simulink model "model_one_upgrade1"  (R2025b)
settings: Solver=VariableStepAuto  StartTime=0.0  StopTime=600  RelTol=1e-3
undefined symbols (not defined in the file or in its folder): battery_builder_rtmsupport, gcbh
libraries: nesl_utility x9, fl_lib x8, Batteries_Pack_lib x2, autolibshared x1, mqttlib x1, batt_lib x1, BatteryBalancing x1
(part 1 of 2)
settings Model: PacingRate=11  Creator=DELL  LastModifiedBy=my802
settings DebuggingCC: AlgebraicLoopMsg=none

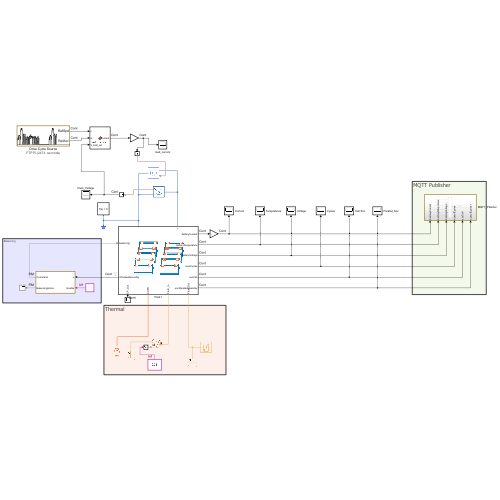
[thumbnail: Simulink's stored preview of the top-level diagram]
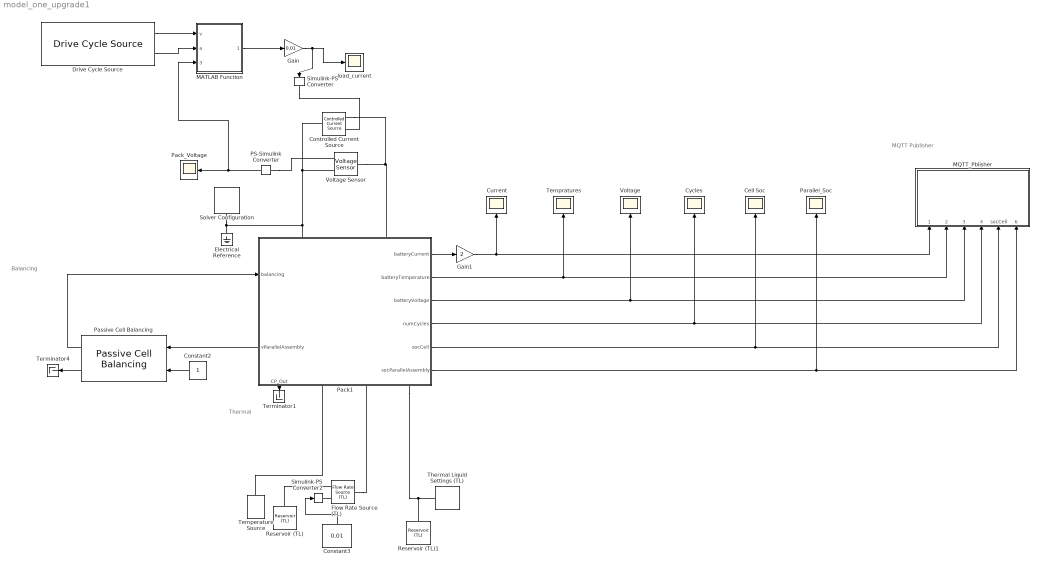
== system model_one_upgrade1 ==
  note: MQTT Publisher
  note: Balancing
  note: Thermal
  Cell Soc : Scope
      settings: ActiveDisplayYMinimum=0.546688606760402  ActiveDisplayYMaximum=0.829439556546784  DataLoggingVariableName=ScopeData6
  Constant2 : Constant
  Constant3 : Constant  Value=0.01
  Controlled Current Source : fl_lib/Electrical/Electrical Sources/Controlled Current Source
  Current : Scope
      settings: ActiveDisplayYMinimum=-32.846312604360023  ActiveDisplayYMaximum=11.836410191491415
  Cycles : Scope
      settings: ActiveDisplayYMinimum=-0.0029468529954673551  ActiveDisplayYMaximum=0.02652167582790381  DataLoggingVariableName=ScopeData9
  Drive Cycle Source : autolibshared/Drive Cycle Source  cycleVar=FTP75  fileVar=cycleFTP75.mat  tfinal="2474  seconds"  cycleRepeat=off  outAccPort=on  outGearPort=off  gearList=No gear data  t_wot1=5  xdot_woto=0  xdot_wot1=30  t_wot2=20  xdot_wot2=0  t_wotend=30  srcUnit=m/s  outUnit=m/s  srcAccUnit=m/s/s  outAccUnit=m/s^2  dt=0  aMode=1  faultOption=off  velBnd=2  velBndUnit=mph  inUnit=m/s  timeBnd=1  failOption=off  stopSim=off  maxFaultCnt=10  maxFaultTime=2  maxTotFaultTime=15  traceOption=off  dtTrace=1  traceWindow=10  lastDCname=FTP75  lastOutUnit=mph  lastDT=0  lastTB=1  lastSB=2  forceCalcBound=off
  Electrical Reference : fl_lib/Electrical/Electrical Elements/Electrical Reference
  Flow Rate Source (TL) : fl_lib/Thermal Liquid/Sources/Flow Rate Source (TL)  source_type=foundation.enum.constant_controlled.controlled  flow_type=foundation.enum.mass_volumetric_flow.mass  mass_flow=0 kg/s  volumetric_flow=0 m^3/s  power_spec=foundation.enum.power_spec.isentropic  area=0.01 m^2
  Gain : Gain  Gain=0.01
  Gain1 : Gain  Gain=2
  MATLAB Function : MATLAB Function  TreatAsAtomicUnit=on
  MQTT_Pblisher : Subsystem
  PS-Simulink Converter : nesl_utility/PS-Simulink Converter  PhysicalDomain=network_engine_domain  SubClassName=ps_output  LeftPortType=input  RightPortType=output  PseudoPeriodic=off  Frequencies=[]  VectorFormat=inherit  Unit=inherit  AffineConversion=off
  Pack1 : Subsystem  LoadFcn=battery_builder_rtmsupport('loadfcn',gcbh);
      settings: CopyFcn=battery_builder_rtmsupport('copyfcn',gcbh);  PreCopyFcn=battery_builder_rtmsupport('precopyfcn',gcbh);  PreDeleteFcn=battery_builder_rtmsupport('predeletefcn',gcbh);  PortSchema="{\"entries\":[{\"content\":{\"sides\":[{\"content\":{\"connectorIds\":[\"LConn1\",\"LConn2\"]},\"type\":\"ConnectorPlacement.EquallySpacedRectSide\",\"uuid\":\"55a5794a-5ecf-4a83-8d77-34dfd6810a2f\"},{\"content\":{\"connectorIds\":[\"Out1\",\"RConn1\",\"RConn2\",\"RConn3\"],\"side\":\"RIGHT\"},\"type\":\"ConnectorPlacement.EquallySpacedRectSide\",\"uuid\":\"d8a6a3e5-5c93-4739-9223-e5221a5356c5\"},{\"content\":{\"connectorIds\":[\"In1\",\"Out8\"],\"side\":\"TOP\"},\"type\":\"ConnectorPlacement.EquallySpacedRectSide\",\"uuid\":\"e9ee7270-cbe6-4e4f-8234-b65e137cf24d\"},{\"content\":{\"connectorIds\":[\"Out2\",\"Out3\",\"Out4\",\"Out5\",\"Out6\",\"Out7\"],\"side\":\"BOTTOM\"},\"type\":\"ConnectorPlacement.EquallySpacedRectSide\",\"uuid\":\"56854e54-bf02-4170-8eb1-11b06e8960f7\"}]},\"type\":\"ConnectorPlacement.EquallySpacedConnector\",\"uuid\":\"e45f6c19-a0f4-4da6-938a-e1e4a4f7821b\"}],\"packageUris\":[\"http://schema.mathworks.com/mf0/Connector/R2020b\"],\"version\":\"1.0\"}"
      mask Display: image('$imagefile')
  Pack_Voltage : Scope
      settings: ActiveDisplayYMinimum=11.015291198745329  ActiveDisplayYMaximum=17.499738477567043
  Parallel_Soc : Scope
      settings: ActiveDisplayYMinimum=0.548996443495374  ActiveDisplayYMaximum=0.8458849402649733  DataLoggingVariableName=ScopeData8
  Passive Cell Balancing : BatteryBalancing/Passive Cell Balancing  Threshold=0.2  HysteresisBand=0  Td_on=1  Td_off=1  Ts=-1  dataType=double
      settings: LibrarySourceBlock=batt_sl_lib/Cell Balancing/Passive Cell Balancing
  Reservoir (TL) : fl_lib/Thermal Liquid/Elements/Reservoir (TL)  pressure_spec=foundation.enum.pressure_spec.atmospheric  reservoir_pressure=0.101325 MPa  reservoir_temperature=293.15 K  area=0.01 m^2
  Reservoir (TL)1 : fl_lib/Thermal Liquid/Elements/Reservoir (TL)  pressure_spec=foundation.enum.pressure_spec.atmospheric  reservoir_pressure=0.101325 MPa  reservoir_temperature=293.15 K  area=0.01 m^2
  Simulink-PS Converter : nesl_utility/Simulink-PS Converter  PhysicalDomain=network_engine_domain  SubClassName=ps_input  LeftPortType=input  RightPortType=output  PseudoPeriodic=off  Frequencies=[]  NoiseDistribution=none  NoiseParameters=[]  Unit=1  AffineConversion=off  FilteringAndDerivatives=provide  SimscapeFilterOrder=1  InputFilterTimeConstant=0.001  UdotUserProvided=0
  Simulink-PS Converter2 : nesl_utility/Simulink-PS Converter  PhysicalDomain=network_engine_domain  SubClassName=ps_input  LeftPortType=input  RightPortType=output  PseudoPeriodic=off  Frequencies=[]  NoiseDistribution=none  NoiseParameters=[]  Unit=1  AffineConversion=off  FilteringAndDerivatives=provide  SimscapeFilterOrder=1  InputFilterTimeConstant=0.001  UdotUserProvided=0
  Solver Configuration : nesl_utility/Solver Configuration  PhysicalDomain=network_engine_domain  SubClassName=solver  LeftPortType=input  RightPortType=generic  Tones=[]  Harmonics=[]  SimulateNoise=off  Profile=off  UseLocalSampling=off  EnableSwitchedLinearOptims=on  FrequencyDomain=off  UseCCode=off  RelTol=0.001  AbsTol=0.001  MinStep=1e-09  ToWorkspace=off  RevertToSquareIcSolve=off  NumHomotopyIterations=100  PhasorMode=off  PhasorModeNumHarmonics=1  ConsistencySolver=NEWTON_XTOL_AFTER_FTOL  IndexReductionMethod=DerivativeReplacement  DoDC=off  ResidualTolerance=1e-09  ConsistencyTolSource=GLOBAL  ConsistencyAbsTol=0.001  ConsistencyRelTol=0.001  ConsistencyTolFactor=0.001  UseLocalSolver=off  LocalSolverChoice=NE_BACKWARD_EULER_ADVANCER  ResolveIndetEquations=on  FunctionEvalNumThread=1  LocalSolverSampleTime=0.001  DoFixedCost=off  MaxNonlinIter=3  MaxModeIter=2  ComputeImpulses=off  ImpulseIterations=2  LinearAlgebra=auto  LinearAlgebraNumThread=0  EquationFormulation=NE_TIME_EF  DelaysMemoryBudget=1024  AutomaticFiltering=on  FilteringTimeConstant=0.001  PartitionStorageMethod=AS_NEEDED  PartitionMemoryBudget=1024  PartitionMethod=ROBUST  MultibodyUseLocalSolver=off  MultibodyLocalSolverChoice=ODE1  MultibodyLocalSolverSampleTime=0.001
  Temperature Source : fl_lib/Thermal/Thermal Sources/Temperature Source  temperature=298.15 K
  Tempratures : Scope
      settings: ActiveDisplayYMinimum=297.03118131262454  ActiveDisplayYMaximum=305.45250178286375  DataLoggingVariableName=ScopeData4
  Terminator1 : Terminator
  Terminator4 : Terminator
  Thermal Liquid Settings (TL) : fl_lib/Thermal Liquid/Utilities/Thermal Liquid Settings (TL)  table_dimensions=foundation.enum.table_dimensions_TL.two_dimensional  T_TLU=[273.1600 : 10 : 373.16]' K  p_TLU=[0.01, 0.1, 5 : 5 : 50] MPa  p_atm=0.101325 MPa  pT_region_flag=foundation.enum.pT_region_TL.min_max  T_min=273.16 K  T_max=373.16 K  p_min=0.01 MPa  p_max=50 MPa  T_min_1D=273.16 K  T_max_1D=373.16 K  p_min_1D=0.01 MPa  p_max_1D=50 MPa  pT_validity_TLU=[1, 1, 1, 1, 1, 1, 1, 1, 1, 1, 1, 1; 1, 1, 1, 1, 1, 1, 1, 1, 1, 1, 1, 1; 1, 1, 1, 1, 1, 1, 1, 1, 1, 1, 1, 1; 1, 1, 1, 1, 1, 1, 1, 1, 1, 1, 1, 1; 1, 1, 1, 1, 1, 1, 1, 1, 1, 1, 1, 1; 0, 1, 1, 1, 1, 1, 1, 1, 1, 1, 1, 1; 0, 1, 1, 1, 1, 1, 1, 1, 1, 1, 1, 1; 0, 1, 1, 1, 1, 1, 1, 1, 1, 1, 1, 1; 0, 1, 1, 1, 1, 1, 1, 1, 1, 1, 1, 1; 0, 1, 1, 1, 1, 1, 1, 1, 1, 1, 1, 1; 0, 0, 1, 1, 1, 1, 1, 1, 1, 1, 1, 1]  properties_range_check=simscape.enum.assert.action.error  rho_parameterization_2D=foundation.enum.rho_parameterization_2D.rho_beta_alpha  rho_parameterization_1D=foundation.enum.rho_parameterization_1D.rho_vector  rho_TLU=[999.7973, 999.8431, 1002.3216, 1004.8218, 1007.293, 1009.7358, 1012.1506, 1014.5379, 1016.8979, 1019.2311, 1021.538, 1023.8188; 999.6579, 999.7009, 1002.0303, 1004.382, 1006.7084, 1009.0101, 1011.2874, 1013.5407, 1015.7703, 1017.9766, 1020.1599, 1022.3206; 998.1632, 998.2045, 1000.4375, 1002.6924, 1004.9239, 1007.1324, 1009.3183, 1011.4819, 1013.6236, 1015.7438, 1017.8428, 1019.921; 995.6057, 995.6458, 997.8186, 1000.0128, 1002.1841, 1004.3332, 1006.4603, 1008.566, 1010.6505, 1012.7144, 1014.758, 1016.7815; 992.1724, 992.2119, 994.3513, 996.5113, 998.6484, 1000.7633, 1002.8563, 1004.928, 1006.9788, 1009.009, 1011.0192, 1013.0097; 988.02, 988.0299, 990.1568, 992.3035, 994.4268, 996.5273, 998.6056, 1000.6622, 1002.6976, 1004.7123, 1006.7067, 1008.6813; 983.18, 983.1901, 985.3217, 987.4721, 989.5983, 991.7008, 993.7803, 995.8374, 997.8726, 999.8864, 1001.8795, 1003.8522; 977.75, 977.7583, 979.9094, 982.0783, 984.2216, 986.34, 988.4343, 990.505, 992.5529, 994.5786, 996.5825, 998.5654; 971.77, 971.7836, 973.9673, 976.1678, 978.3409, 980.4876, 982.6087, 984.7049, 986.7768, 988.8254, 990.8511, 992.8545; 965.26, 965.3023, 967.5311, 969.7753, 971.9901, 974.1764, 976.3354, 978.4676, 980.5741, 982.6556, 984.7129, 986.7465; 958.62, 958.6315, 960.627, 962.9267, 965.1944, 967.4314, 969.6387, 971.8173, 973.9681, 976.0921, 978.19, 980.2628] kg/m^3  beta_TLU=[1.9649, 1.9654, 1.9929, 2.0213, 2.0499, 2.0787, 2.1078, 2.1372, 2.1668, 2.1966, 2.2268, 2.2572; 2.0913, 2.0918, 2.1191, 2.1471, 2.1752, 2.2036, 2.2322, 2.261, 2.2899, 2.3191, 2.3485, 2.3781; 2.1786, 2.1791, 2.2067, 2.235, 2.2634, 2.2919, 2.3206, 2.3494, 2.3784, 2.4075, 2.4367, 2.4661; 2.2332, 2.2337, 2.2619, 2.2908, 2.3197, 2.3487, 2.3778, 2.407, 2.4363, 2.4657, 2.4951, 2.5246; 2.26, 2.2605, 2.2895, 2.3191, 2.3487, 2.3784, 2.4081, 2.4378, 2.4675, 2.4973, 2.5272, 2.5571; 2.2638, 2.2638, 2.2936, 2.324, 2.3544, 2.3848, 2.4151, 2.4455, 2.4758, 2.5062, 2.5365, 2.5669; 2.2472, 2.2472, 2.2779, 2.3092, 2.3403, 2.3715, 2.4025, 2.4336, 2.4646, 2.4955, 2.5264, 2.5573; 2.214, 2.214, 2.2455, 2.2776, 2.3096, 2.3415, 2.3733, 2.405, 2.4367, 2.4683, 2.4998, 2.5313; 2.1668, 2.1668, 2.1992, 2.2321, 2.2649, 2.2976, 2.3301, 2.3626, 2.3949, 2.4272, 2.4593, 2.4914; 2.1081, 2.1081, 2.1413, 2.175, 2.2086, 2.2421, 2.2754, 2.3085, 2.3415, 2.3744, 2.4072, 2.4399; 2.0494, 2.0494, 2.0739, 2.1084, 2.1428, 2.177, 2.211, 2.2449, 2.2786, 2.3121, 2.3455, 2.3788] GPa  alpha_TLU=1e-4 * [-.679, -.676, -.49, -.307, -.13, .041, .206, .365, .519, .668, .811, .949; .878, .881, .998, 1.114, 1.227, 1.337, 1.445, 1.549, 1.651, 1.75, 1.846, 1.939; 2.068, 2.069, 2.141, 2.213, 2.283, 2.352, 2.42, 2.486, 2.551, 2.614, 2.676, 2.736; 3.034, 3.035, 3.074, 3.113, 3.152, 3.191, 3.229, 3.267, 3.305, 3.341, 3.377, 3.413; 3.855, 3.856, 3.87, 3.884, 3.899, 3.914, 3.93, 3.946, 3.961, 3.977, 3.993, 4.009; 4.578, 4.578, 4.572, 4.566, 4.562, 4.558, 4.555, 4.552, 4.55, 4.549, 4.548, 4.547; 5.233, 5.233, 5.209, 5.186, 5.165, 5.144, 5.125, 5.107, 5.09, 5.074, 5.059, 5.045; 5.84, 5.84, 5.801, 5.762, 5.725, 5.691, 5.657, 5.625, 5.595, 5.566, 5.538, 5.512; 6.414, 6.414, 6.36, 6.307, 6.256, 6.208, 6.161, 6.117, 6.074, 6.033, 5.994, 5.956; 6.967, 6.967, 6.898, 6.831, 6.766, 6.705, 6.646, 6.589, 6.535, 6.482, 6.432, 6.384; 7.519, 7.519, 7.423, 7.342, 7.264, 7.189, 7.118, 7.049, 6.983, 6.92, 6.859, 6.8] 1/K  rho_TLU_2=[999.7973, 999.8431, 1002.3216, 1004.8218, 1007.293, 1009.7358, 1012.1506, 1014.5379, 1016.8979, 1019.2311, 1021.538, 1023.8188; 999.6579, 999.7009, 1002.0303, 1004.382, 1006.7084, 1009.0101, 1011.2874, 1013.5407, 1015.7703, 1017.9766, 1020.1599, 1022.3206; 998.1632, 998.2045, 1000.4375, 1002.6924, 1004.9239, 1007.1324, 1009.3183, 1011.4819, 1013.6236, 1015.7438, 1017.8428, 1019.921; 995.6057, 995.6458, 997.81864, 1000.0128, 1002.1841, 1004.3332, 1006.4603, 1008.566, 1010.6505, 1012.7144, 1014.758, 1016.7815; 992.1724, 992.2119, 994.3513, 996.5113, 998.6484, 1000.7633, 1002.8563, 1004.928, 1006.9788, 1009.009, 1011.0192, 1013.0097; 988.02, 988.0299, 990.1568, 992.3035, 994.4268, 996.5273, 998.6056, 1000.6622, 1002.6976, 1004.7123, 1006.7067, 1008.6813; 983.18, 983.1901, 985.3217, 987.4721, 989.5983, 991.7008, 993.7803, 995.8374, 997.8726, 999.8864, 1001.8795, 1003.8522; 977.75, 977.7583, 979.9094, 982.0783, 984.2216, 986.34, 988.4343, 990.505, 992.5529, 994.5786, 996.5825, 998.5654; 971.77, 971.7836, 973.9673, 976.1678, 978.3409, 980.4876, 982.6087, 984.7049, 986.7768, 988.8254, 990.8511, 992.8545; 965.26, 965.3023, 967.5311, 969.7753, 971.9901, 974.1764, 976.3354, 978.4676, 980.5741, 982.6556, 984.7129, 986.7465; 958.62, 958.6315, 960.627, 962.9267, 965.1944, 967.4314, 969.6387, 971.8173, 973.9681, 976.0921, 978.19, 980.2628] kg/m^3  rho_ref_3=998.21 kg/m^3  T_ref_3=293.16 K  p_ref_3=0.101325 MPa  beta_const_3=2.1791 GPa  alpha_const_3=2.0691e-4 1/K  rho_TLU_4=[999.84; 999.7; 998.2; 995.65; 992.21; 988.03; 983.19; 977.76; 971.78; 965.3; 958.8] kg/m^3  beta_const_4=2.1791 GPa  p_ref_4=0.101325 MPa  rho_ref_5=998.21 kg/m^3  T_ref_5=293.16 K  p_ref_5=0.101325 MPa  beta_const_5=2.1791 GPa  alpha_const_5=2.0691e-4 1/K  u_parameterization_2D=foundation.enum.u_parameterization_2D.u_cp  u_parameterization_1D=foundation.enum.u_parameterization_1D.u  u_TLU=[.0002, .0018, .086, .1588, .219, .267, .3034, .3288, .3436, .3483, .3435, .3294; 42.062, 42.06, 41.935, 41.804, 41.668, 41.527, 41.382, 41.233, 41.081, 40.924, 40.763, 40.599; 83.953, 83.948, 83.651, 83.349, 83.049, 82.749, 82.451, 82.153, 81.856, 81.56, 81.265, 80.971; 125.77, 125.76, 125.31, 124.86, 124.41, 123.97, 123.53, 123.1, 122.68, 122.25, 121.84, 121.42; 167.57, 167.56, 166.96, 166.37, 165.79, 165.21, 164.65, 164.09, 163.54, 163, 162.46, 161.94; 209.36, 209.36, 208.63, 207.9, 207.19, 206.48, 205.79, 205.11, 204.45, 203.79, 203.14, 202.5; 251.19, 251.19, 250.33, 249.47, 248.62, 247.79, 246.98, 246.18, 245.39, 244.62, 243.86, 243.12; 293.06, 293.06, 292.07, 291.07, 290.1, 289.14, 288.2, 287.28, 286.38, 285.49, 284.62, 283.77; 334.99, 334.99, 333.86, 332.73, 331.63, 330.54, 329.48, 328.44, 327.41, 326.41, 325.43, 324.46; 377, 377, 375.73, 374.46, 373.22, 372, 370.81, 369.64, 368.5, 367.38, 366.27, 365.19; 419.01, 419.01, 417.69, 416.27, 414.89, 413.54, 412.21, 410.91, 409.64, 408.4, 407.17, 405.98] kJ/kg  cp_TLU=[4.2199, 4.2194, 4.1957, 4.1726, 4.1508, 4.13, 4.1103, 4.0916, 4.0738, 4.0569, 4.0408, 4.0254; 4.1955, 4.1951, 4.1769, 4.1592, 4.1422, 4.1259, 4.1103, 4.0954, 4.0812, 4.0676, 4.0545, 4.0421; 4.1843, 4.184, 4.169, 4.1543, 4.1401, 4.1264, 4.1133, 4.1007, 4.0885, 4.0768, 4.0656, 4.0548; 4.1801, 4.1798, 4.1667, 4.1538, 4.1413, 4.1293, 4.1177, 4.1064, 4.0956, 4.0851, 4.075, 4.0653; 4.1796, 4.1794, 4.1675, 4.1558, 4.1444, 4.1334, 4.1227, 4.1123, 4.1023, 4.0926, 4.0832, 4.0741; 4.1813, 4.1813, 4.1702, 4.1592, 4.1484, 4.138, 4.1279, 4.1181, 4.1086, 4.0993, 4.0903, 4.0816; 4.185, 4.185, 4.1742, 4.1636, 4.1532, 4.1432, 4.1334, 4.1239, 4.1146, 4.1056, 4.0969, 4.0884; 4.1901, 4.1901, 4.1795, 4.169, 4.1588, 4.1489, 4.1393, 4.1299, 4.1207, 4.1118, 4.1032, 4.0947; 4.1968, 4.1968, 4.1862, 4.1757, 4.1655, 4.1555, 4.1458, 4.1364, 4.1273, 4.1183, 4.1096, 4.1012; 4.2052, 4.2052, 4.1944, 4.1837, 4.1733, 4.1632, 4.1534, 4.1438, 4.1345, 4.1255, 4.1166, 4.108; 4.2136, 4.2136, 4.2045, 4.1935, 4.1828, 4.1724, 4.1623, 4.1524, 4.1429, 4.1335, 4.1245, 4.1157] kJ/(K*kg)  u_TLU_2=[.0002, .0018, .086, .1588, .219, .267, .3034, .3288, .3436, .3483, .3435, .3294; 42.062, 42.06, 41.935, 41.804, 41.668, 41.527, 41.382, 41.233, 41.081, 40.924, 40.763, 40.599; 83.953, 83.948, 83.651, 83.349, 83.049, 82.749, 82.451, 82.153, 81.856, 81.56, 81.265, 80.971; 125.77, 125.76, 125.31, 124.86, 124.41, 123.97, 123.53, 123.1, 122.68, 122.25, 121.84, 121.42; 167.57, 167.56, 166.96, 166.37, 165.79, 165.21, 164.65, 164.09, 163.54, 163, 162.46, 161.94; 209.36, 209.36, 208.63, 207.9, 207.19, 206.48, 205.79, 205.11, 204.45, 203.79, 203.14, 202.5; 251.19, 251.19, 250.33, 249.47, 248.62, 247.79, 246.98, 246.18, 245.39, 244.62, 243.86, 243.12; 293.06, 293.06, 292.07, 291.07, 290.1, 289.14, 288.2, 287.28, 286.38, 285.49, 284.62, 283.77; 334.99, 334.99, 333.86, 332.73, 331.63, 330.54, 329.48, 328.44, 327.41, 326.41, 325.43, 324.46; 377, 377, 375.73, 374.46, 373.22, 372, 370.81, 369.64, 368.5, 367.38, 366.27, 365.19; 419.01, 419.01, 417.69, 416.27, 414.89, 413.54, 412.21, 410.91, 409.64, 408.4, 407.17, 405.98] kJ/kg  cp_TLU_3=[4.2199, 4.2194, 4.1957, 4.1726, 4.1508, 4.13, 4.1103, 4.0916, 4.0738, 4.0569, 4.0408, 4.0254; 4.1955, 4.1951, 4.1769, 4.1592, 4.1422, 4.1259, 4.1103, 4.0954, 4.0812, 4.0676, 4.0545, 4.0421; 4.1843, 4.184, 4.169, 4.1543, 4.1401, 4.1264, 4.1133, 4.1007, 4.0885, 4.0768, 4.0656, 4.0548; 4.1801, 4.1798, 4.1667, 4.1538, 4.1413, 4.1293, 4.1177, 4.1064, 4.0956, 4.0851, 4.075, 4.0653; 4.1796, 4.1794, 4.1675, 4.1558, 4.1444, 4.1334, 4.1227, 4.1123, 4.1023, 4.0926, 4.0832, 4.0741; 4.1813, 4.1813, 4.1702, 4.1592, 4.1484, 4.138, 4.1279, 4.1181, 4.1086, 4.0993, 4.0903, 4.0816; 4.185, 4.185, 4.1742, 4.1636, 4.1532, 4.1432, 4.1334, 4.1239, 4.1146, 4.1056, 4.0969, 4.0884; 4.1901, 4.1901, 4.1795, 4.169, 4.1588, 4.1489, 4.1393, 4.1299, 4.1207, 4.1118, 4.1032, 4.0947; 4.1968, 4.1968, 4.1862, 4.1757, 4.1655, 4.1555, 4.1458, 4.1364, 4.1273, 4.1183, 4.1096, 4.1012; 4.2052, 4.2052, 4.1944, 4.1837, 4.1733, 4.1632, 4.1534, 4.1438, 4.1345, 4.1255, 4.1166, 4.108; 4.2136, 4.2136, 4.2045, 4.1935, 4.1828, 4.1724, 4.1623, 4.1524, 4.1429, 4.1335, 4.1245, 4.1157] kJ/(K*kg)  u_TLU_4=[.0018; 42.06; 83.948; 125.76; 167.56; 209.36; 251.19; 293.06; 334.99; 377; 418.01] kJ/kg  cp_TLU_5=[4.2199; 4.1955; 4.1843; 4.1801; 4.1796; 4.1813; 4.185; 4.1901; 4.1968; 4.2052; 4.2136] kJ/(K*kg)  nu_TLU=[1.7917, 1.7914, 1.7763, 1.7615, 1.7473, 1.7338, 1.7208, 1.7085, 1.6967, 1.6854, 1.6747, 1.6645; 1.3061, 1.3059, 1.2986, 1.2914, 1.2845, 1.2779, 1.2716, 1.2656, 1.2598, 1.2543, 1.2491, 1.2441; 1.0032, 1.0032, .9995, .9959, .9924, .9891, .9859, .9829, .9801, .9774, .9748, .9724; .8006, .8005, .7987, .797, .7953, .7937, .7922, .7908, .7894, .7881, .787, .7859; .6577, .6577, .657, .6562, .6555, .6548, .6543, .6537, .6532, .6528, .6523, .652; .553, .553, .5529, .5527, .5526, .5525, .5524, .5524, .5524, .5524, .5524, .5525; .4739, .4739, .4741, .4743, .4745, .4747, .475, .4753, .4755, .4758, .4762, .4765; .4127, .4127, .4131, .4135, .4139, .4143, .4148, .4152, .4157, .4162, .4167, .4172; .3643, .3643, .3648, .3654, .3659, .3665, .367, .3676, .3682, .3688, .3694, .37; .3254, .3254, .3261, .3267, .3273, .328, .3286, .3293, .3299, .3306, .3312, .3319; .2866, .2866, .2945, .2952, .2959, .2965, .2972, .2979, .2986, .2993, .3, .3007] mm^2/s  nu_TLU_2=[1.7917; 1.3061; 1.0032; .8006; .6577; .553; .4739; .4127; .3643; .3254; .2866] mm^2/s  k_TLU=[561.04, 561.09, 563.8, 566.56, 569.32, 572.08, 574.82, 577.54, 580.24, 582.92, 585.57, 588.18; 580.02, 580.07, 582.45, 584.88, 587.32, 589.75, 592.18, 594.61, 597.02, 599.42, 601.8, 604.16; 598.44, 598.48, 600.73, 603.03, 605.33, 607.64, 609.94, 612.24, 614.54, 616.82, 619.1, 621.36; 615.48, 615.52, 617.73, 620, 622.26, 624.54, 626.81, 629.07, 631.34, 633.6, 635.85, 638.09; 630.6, 630.64, 632.87, 635.15, 637.44, 639.72, 642.01, 644.29, 646.57, 648.84, 651.11, 653.36; 643.61, 643.61, 645.88, 648.21, 650.53, 652.86, 655.18, 657.51, 659.82, 662.14, 664.44, 666.74; 654.39, 654.39, 656.73, 659.12, 661.5, 663.89, 666.27, 668.65, 671.02, 673.38, 675.74, 678.09; 663.13, 663.13, 665.54, 668, 670.46, 672.91, 675.36, 677.8, 680.24, 682.67, 685.09, 687.5; 670.02, 670.02, 672.51, 675.05, 677.59, 680.12, 682.64, 685.16, 687.67, 690.17, 692.66, 695.14; 675.27, 675.27, 677.85, 680.48, 683.11, 685.73, 688.34, 690.94, 693.53, 696.11, 698.68, 701.24; 680.52, 680.52, 681.77, 684.5, 687.22, 689.94, 692.64, 695.34, 698.02, 700.69, 703.35, 706] mW/(K*m)  k_TLU_2=[561.04; 580.02; 598.44; 615.48; 630.6; 643.61; 654.39; 663.13; 670.02; 675.27; 680.52] mW/(K*m)
  Voltage : Scope
      settings: ActiveDisplayYMinimum=3.7175558325329772  ActiveDisplayYMaximum=4.5563975278034681  DataLoggingVariableName=ScopeData5
  Voltage Sensor : fl_lib/Electrical/Electrical Sensors/Voltage Sensor
  load_current : Scope
      settings: ActiveDisplayYMinimum=-11.836404348489875  ActiveDisplayYMaximum=32.8462600292936  DataLoggingVariableName=ScopeData2
  wires:
  Constant2/1 -> Passive Cell Balancing/2
  Pack1/8(vParallelAssembly) -> Passive Cell Balancing/1
  Pack1/1(CP_Out) -> Terminator1/1
  Pack1/7(socParallelAssembly) -> Parallel_Soc/1, MQTT_Pblisher/6(numofCycles1)
  Pack1/5(numCycles) -> Cycles/1, MQTT_Pblisher/4(numofCycles)
  Pack1/4(batteryVoltage) -> Voltage/1, MQTT_Pblisher/3(batteryVoltage)
  Pack1/3(batteryTemperature) -> Tempratures/1, MQTT_Pblisher/2(batteryTemprature)
  Passive Cell Balancing/2 -> Terminator4/1
  Constant3/1 -> Simulink-PS Converter2/1
  Passive Cell Balancing/1 -> Pack1/1(balancing)
  Pack1/6(socCell) -> Cell Soc/1, MQTT_Pblisher/5(socCell)
  Drive Cycle Source/1 -> MATLAB Function/1(v)
  Drive Cycle Source/2 -> MATLAB Function/2(a)
  PS-Simulink Converter/1 -> Pack_Voltage/1, MATLAB Function/3(V_batt_act)
  MATLAB Function/1(Current) -> Gain/1
  Gain/1 -> Simulink-PS Converter/1, load_current/1
  Pack1/2(batteryCurrent) -> Gain1/1
  Gain1/1 -> MQTT_Pblisher/1(batteryCurrent), Current/1
  connections:
  Solver Configuration/RConn1 -- Voltage Sensor/RConn2 -- Controlled Current Source/LConn1 -- Pack1/LConn1 -- Electrical Reference/LConn1
  Reservoir (TL)/LConn1 -- Flow Rate Source (TL)/LConn1
  Flow Rate Source (TL)/RConn1 -- Pack1/RConn2
  Pack1/RConn3 -- Thermal Liquid Settings (TL)/RConn1 -- Reservoir (TL)1/LConn1
  Temperature Source/LConn1 -- Pack1/RConn1
  Simulink-PS Converter2/RConn1 -- Flow Rate Source (TL)/LConn2
  Voltage Sensor/LConn1 -- Controlled Current Source/RConn2 -- Pack1/LConn2
  PS-Simulink Converter/LConn1 -- Voltage Sensor/RConn1
  Simulink-PS Converter/RConn1 -- Controlled Current Source/RConn1

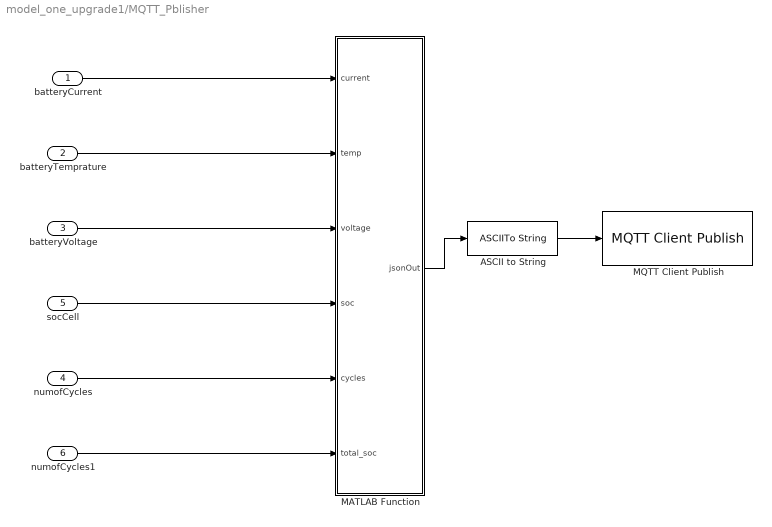
== system model_one_upgrade1/MQTT_Pblisher ==
  batteryCurrent : Inport
  batteryTemprature : Inport  Port=2
  batteryVoltage : Inport  Port=3
  numofCycles : Inport  Port=4
  socCell : Inport  Port=5
  numofCycles1 : Inport  Port=6
  ASCII to String : ASCIIToString
  MATLAB Function : MATLAB Function  TreatAsAtomicUnit=on
  MQTT Client Publish : mqttlib/MQTT Client Publish  RetainClient=MQTT_BROKER  ClientList=MQTT_BROKER  TopicsTable={ '1', 'Pack', '0', 'on' }  PublishOnDataChange=on  SampleTime=-1  TopicNames=Pack  NumTopics=1  IsLib=0  BlkName=MQTT Client Publish
  wires:
  batteryCurrent/1 -> MATLAB Function/1(current)
  batteryTemprature/1 -> MATLAB Function/2(temp)
  batteryVoltage/1 -> MATLAB Function/3(voltage)
  numofCycles/1 -> MATLAB Function/5(cycles)
  socCell/1 -> MATLAB Function/4(soc)
  MATLAB Function/1(jsonOut) -> ASCII to String/1
  ASCII to String/1 -> MQTT Client Publish/1
  numofCycles1/1 -> MATLAB Function/6(total_soc)

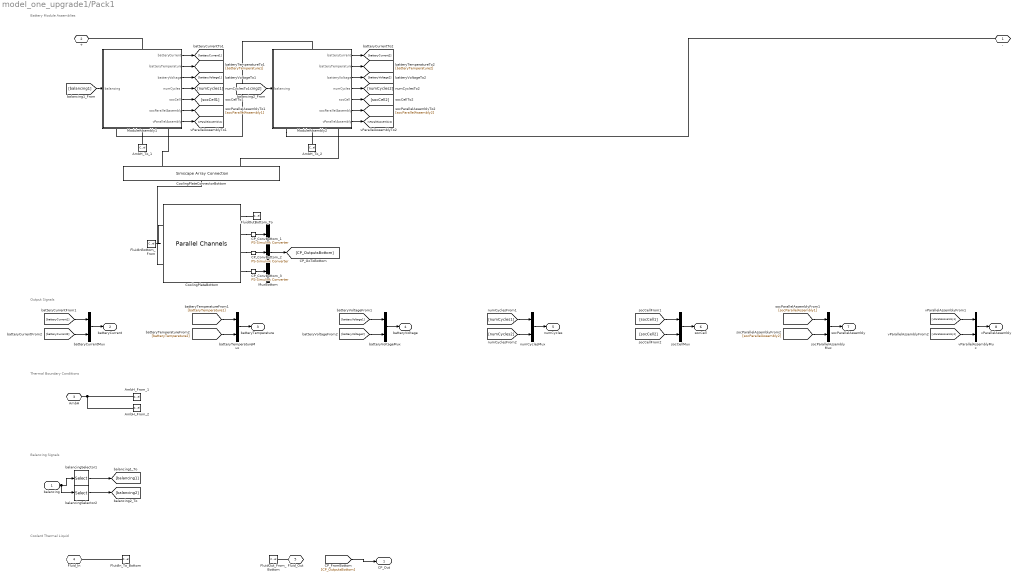
== system model_one_upgrade1/Pack1 ==
  note: Coolant Thermal Liquid
  note: Balancing Signals
  note: Thermal Boundary Conditions
  note: Output Signals
  note: Battery Module Assemblies
  balancing : Inport  PortDimensions=4
  AmbH_From_1 : ConnectionLabel  Label=ambH_1
  AmbH_From_2 : ConnectionLabel  Label=ambH_2
  AmbH_To_1 : ConnectionLabel  Label=ambH_1
  AmbH_To_2 : ConnectionLabel  Label=ambH_2
  CP_ConvBottom_1 : nesl_utility/PS-Simulink Converter  PhysicalDomain=network_engine_domain  SubClassName=ps_output  LeftPortType=input  RightPortType=output  PseudoPeriodic=off  Frequencies=[]  VectorFormat=inherit  Unit=inherit  AffineConversion=off
  CP_ConvBottom_2 : nesl_utility/PS-Simulink Converter  PhysicalDomain=network_engine_domain  SubClassName=ps_output  LeftPortType=input  RightPortType=output  PseudoPeriodic=off  Frequencies=[]  VectorFormat=inherit  Unit=inherit  AffineConversion=off
  CP_ConvBottom_3 : nesl_utility/PS-Simulink Converter  PhysicalDomain=network_engine_domain  SubClassName=ps_output  LeftPortType=input  RightPortType=output  PseudoPeriodic=off  Frequencies=[]  VectorFormat=inherit  Unit=inherit  AffineConversion=off
  CoolingPlateBottom : batt_lib/Thermal/Parallel Channels  plateConnectivity=simscape.battery.enum.thermal.coolingPlateConnectivity.singleSided  numBattThermalNodes1=8  dimensionThermalNodes1=[[0.02 0.02;0.02 0.02;0.02 0.02;0.02 0.02;0.02 0.02;0.02 0.02;0.02 0.02;0.02 0.02]]  locationThermalNodes1=[[0.01 0.01;0.031 0.01;0.01 0.031;0.031 0.031;0.052 0.01;0.073 0.01;0.052 0.031;0.073 0.031]]  numBattThermalNodes2=1  dimensionThermalNodes2=ones(1, 2)  locationThermalNodes2=ones(1, 2)  plateDimX=2  plateDimY=5  plateTh=2e-3 m  plateThCond=20 W/(K*m)  plateDen=2500 kg/m^3  plateCp=447 J/(K*kg)  plateTemp_ini=300 K  Re_lam=2000  Re_tur=4000  Nu_lam=3.66  length_add=1e-3 m  shape_factor=64  nChannels=4  selectChannelOrientation=simscape.battery.enum.thermal.coolingChannelsDirection.alongX  channelDia=0.005 m  distributorDia=0.005 m  roughnessPipe=1.5e-05 m
      settings: InternalSimscapePortConfiguration="{\"Bottom\":[],\"Left\":[{\"id\":\"fluid_in\",\"label\":\"fluid_in\",\"type\":\"foundation.thermal_liquid.thermal_liquid\"}],\"Right\":[{\"id\":\"fluid_out\",\"label\":\"fluid_out\",\"type\":\"foundation.thermal_liquid.thermal_liquid\"},{\"id\":\"plotPlateT\",\"label\":\"Tp\",\"type\":\"output\"},{\"id\":\"tempSensor\",\"label\":\"dT\",\"type\":\"output\"},{\"id\":\"presSensor\",\"label\":\"dP\",\"type\":\"output\"}],\"Top\":[{\"id\":\"Side1\",\"label\":\"Surf1\",\"type\":\"foundation.thermal.thermal\"}]}"
  CoolingPlateConnectorBottom : SimscapeArrayConnection  Domain=foundation.thermal.thermal  Mode=Sized Elements
  FluidInBottom_From : ConnectionLabel  Label=FluidIn_To_Bottom
  FluidIn_To_Bottom : ConnectionLabel  Label=FluidIn_To_Bottom
  FluidOutBottom_To : ConnectionLabel  Label=FluidOut_From_Bottom
  FluidOut_From_Bottom : ConnectionLabel  Label=FluidOut_From_Bottom
  ModuleAssembly1 : Subsystem  LoadFcn=battery_builder_rtmsupport('loadfcn',gcbh);
      settings: CopyFcn=battery_builder_rtmsupport('copyfcn',gcbh);  PreCopyFcn=battery_builder_rtmsupport('precopyfcn',gcbh);  PreDeleteFcn=battery_builder_rtmsupport('predeletefcn',gcbh);  PortSchema="{\"entries\":[{\"content\":{\"sides\":[{\"content\":{\"connectorIds\":[\"LConn1\"]},\"type\":\"ConnectorPlacement.EquallySpacedRectSide\",\"uuid\":\"95d21288-1122-4a9c-9db4-7a3a66bbb9a8\"},{\"content\":{\"connectorIds\":[\"RConn1\",\"RConn2\",\"RConn3\"],\"side\":\"RIGHT\"},\"type\":\"ConnectorPlacement.EquallySpacedRectSide\",\"uuid\":\"521fc822-c83f-4262-8b01-b075edee4de7\"},{\"content\":{\"connectorIds\":[\"In1\"],\"side\":\"TOP\"},\"type\":\"ConnectorPlacement.EquallySpacedRectSide\",\"uuid\":\"6803cc33-38c7-4653-9a94-590f2e2b7a9a\"},{\"content\":{\"connectorIds\":[\"Out1\",\"Out2\",\"Out3\",\"Out4\",\"Out5\",\"Out6\",\"Out7\"],\"side\":\"BOTTOM\"},\"type\":\"ConnectorPlacement.EquallySpacedRectSide\",\"uuid\":\"5a0984a0-8440-4621-aa61-9d5ed27b7c7c\"}]},\"type\":\"ConnectorPlacement.EquallySpacedConnector\",\"uuid\":\"262ef02e-51cf-43c8-a01c-3c94ee79f83d\"}],\"packageUris\":[\"http://schema.mathworks.com/mf0/Connector/R2020b\"],\"version\":\"1.0\"}"
      mask Display: image('$imagefile')
  ModuleAssembly2 : Subsystem  LoadFcn=battery_builder_rtmsupport('loadfcn',gcbh);
      settings: CopyFcn=battery_builder_rtmsupport('copyfcn',gcbh);  PreCopyFcn=battery_builder_rtmsupport('precopyfcn',gcbh);  PreDeleteFcn=battery_builder_rtmsupport('predeletefcn',gcbh);  PortSchema="{\"entries\":[{\"content\":{\"sides\":[{\"content\":{\"connectorIds\":[\"LConn1\"]},\"type\":\"ConnectorPlacement.EquallySpacedRectSide\",\"uuid\":\"95d21288-1122-4a9c-9db4-7a3a66bbb9a8\"},{\"content\":{\"connectorIds\":[\"RConn1\",\"RConn2\",\"RConn3\"],\"side\":\"RIGHT\"},\"type\":\"ConnectorPlacement.EquallySpacedRectSide\",\"uuid\":\"521fc822-c83f-4262-8b01-b075edee4de7\"},{\"content\":{\"connectorIds\":[\"In1\"],\"side\":\"TOP\"},\"type\":\"ConnectorPlacement.EquallySpacedRectSide\",\"uuid\":\"6803cc33-38c7-4653-9a94-590f2e2b7a9a\"},{\"content\":{\"connectorIds\":[\"Out1\",\"Out2\",\"Out3\",\"Out4\",\"Out5\",\"Out6\",\"Out7\"],\"side\":\"BOTTOM\"},\"type\":\"ConnectorPlacement.EquallySpacedRectSide\",\"uuid\":\"5a0984a0-8440-4621-aa61-9d5ed27b7c7c\"}]},\"type\":\"ConnectorPlacement.EquallySpacedConnector\",\"uuid\":\"262ef02e-51cf-43c8-a01c-3c94ee79f83d\"}],\"packageUris\":[\"http://schema.mathworks.com/mf0/Connector/R2020b\"],\"version\":\"1.0\"}"
      mask Display: image('moduleAssembly_1.JPG');
  MuxBottom : Mux  Inputs=3
  balancingSelector1 : Selector  InputPortWidth=4  IndexOptions=Index vector (dialog)  Indices="[1  2]"  OutputSizes=1
  balancingSelector2 : Selector  InputPortWidth=4  IndexOptions=Index vector (dialog)  Indices="[3  4]"  OutputSizes=1
  batteryCurrentMux : Mux  Inputs=2
  batteryTemperatureMux : Mux  Inputs=2
  batteryVoltageMux : Mux  Inputs=2
  numCyclesMux : Mux  Inputs=2
  socCellMux : Mux  Inputs=2
  socParallelAssemblyMux : Mux  Inputs=2
  vParallelAssemblyMux : Mux  Inputs=2
  - : PMIOPort  Side=Left
  + : PMIOPort  Port=2  Side=Left
  AmbH : PMIOPort  Port=3  Side=Right  ConnectionType=Connection: foundation.thermal.thermal
  Fluid_In : PMIOPort  Port=4  Side=Right  ConnectionType=Connection: foundation.thermal_liquid.thermal_liquid
  Fluid_Out : PMIOPort  Port=5  Side=Right  ConnectionType=Connection: foundation.thermal_liquid.thermal_liquid
  CP_Out : Outport
  batteryCurrent : Outport  Port=2
  batteryTemperature : Outport  Port=3
  batteryVoltage : Outport  Port=4
  numCycles : Outport  Port=5
  socCell : Outport  Port=6
  socParallelAssembly : Outport  Port=7
  vParallelAssembly : Outport  Port=8
  wires:
  [CP_OutputsBottom] -> CP_Out/1
  MuxBottom/1 -> [CP_OutputsBottom]
  CP_ConvBottom_3/1 -> MuxBottom/3
  CP_ConvBottom_2/1 -> MuxBottom/2
  CP_ConvBottom_1/1 -> MuxBottom/1
  balancingSelector2/1 -> [balancing2]
  [balancing2] -> ModuleAssembly2/1(balancing)
  balancingSelector1/1 -> [balancing1]
  balancing/1 -> balancingSelector2/1, balancingSelector1/1
  [balancing1] -> ModuleAssembly1/1(balancing)
  [vParallelAssembly2] -> vParallelAssemblyMux/2
  ModuleAssembly2/7(vParallelAssembly) -> [vParallelAssembly2]
  [socParallelAssembly2] -> socParallelAssemblyMux/2
  ModuleAssembly2/6(socParallelAssembly) -> [socParallelAssembly2]
  [socCell2] -> socCellMux/2
  ModuleAssembly2/5(socCell) -> [socCell2]
  [numCycles2] -> numCyclesMux/2
  ModuleAssembly2/4(numCycles) -> [numCycles2]
  [batteryVoltage2] -> batteryVoltageMux/2
  ModuleAssembly2/3(batteryVoltage) -> [batteryVoltage2]
  [batteryTemperature2] -> batteryTemperatureMux/2
  ModuleAssembly2/2(batteryTemperature) -> [batteryTemperature2]
  [batteryCurrent2] -> batteryCurrentMux/2
  ModuleAssembly2/1(batteryCurrent) -> [batteryCurrent2]
  [vParallelAssembly1] -> vParallelAssemblyMux/1
  vParallelAssemblyMux/1 -> vParallelAssembly/1
  ModuleAssembly1/7(vParallelAssembly) -> [vParallelAssembly1]
  [socParallelAssembly1] -> socParallelAssemblyMux/1
  socParallelAssemblyMux/1 -> socParallelAssembly/1
  ModuleAssembly1/6(socParallelAssembly) -> [socParallelAssembly1]
  [socCell1] -> socCellMux/1
  socCellMux/1 -> socCell/1
  ModuleAssembly1/5(socCell) -> [socCell1]
  [numCycles1] -> numCyclesMux/1
  numCyclesMux/1 -> numCycles/1
  ModuleAssembly1/4(numCycles) -> [numCycles1]
  [batteryVoltage1] -> batteryVoltageMux/1
  batteryVoltageMux/1 -> batteryVoltage/1
  ModuleAssembly1/3(batteryVoltage) -> [batteryVoltage1]
  [batteryTemperature1] -> batteryTemperatureMux/1
  batteryTemperatureMux/1 -> batteryTemperature/1
  ModuleAssembly1/2(batteryTemperature) -> [batteryTemperature1]
  [batteryCurrent1] -> batteryCurrentMux/1
  batteryCurrentMux/1 -> batteryCurrent/1
  ModuleAssembly1/1(batteryCurrent) -> [batteryCurrent1]
  connections:
  CoolingPlateBottom/RConn4 -- CP_ConvBottom_3/LConn1
  CoolingPlateBottom/RConn3 -- CP_ConvBottom_2/LConn1
  CoolingPlateBottom/RConn2 -- CP_ConvBottom_1/LConn1
  CoolingPlateBottom/RConn1 -- FluidOutBottom_To/LConn1
  FluidInBottom_From/LConn1 -- CoolingPlateBottom/LConn1
  Fluid_Out/RConn1 -- FluidOut_From_Bottom/LConn1
  FluidIn_To_Bottom/LConn1 -- Fluid_In/RConn1
  CoolingPlateConnectorBottom/RConn1 -- CoolingPlateBottom/LConn2
  CoolingPlateConnectorBottom/LConn2 -- ModuleAssembly2/RConn3
  CoolingPlateConnectorBottom/LConn1 -- ModuleAssembly1/RConn3
  AmbH_To_2/LConn1 -- ModuleAssembly2/RConn2
  AmbH_From_2/LConn1 -- AmbH_From_1/LConn1 -- AmbH/RConn1
  AmbH_To_1/LConn1 -- ModuleAssembly1/RConn2
  ModuleAssembly2/RConn1 -- -/RConn1
  ModuleAssembly1/LConn1 -- +/RConn1
  ModuleAssembly2/LConn1 -- ModuleAssembly1/RConn1

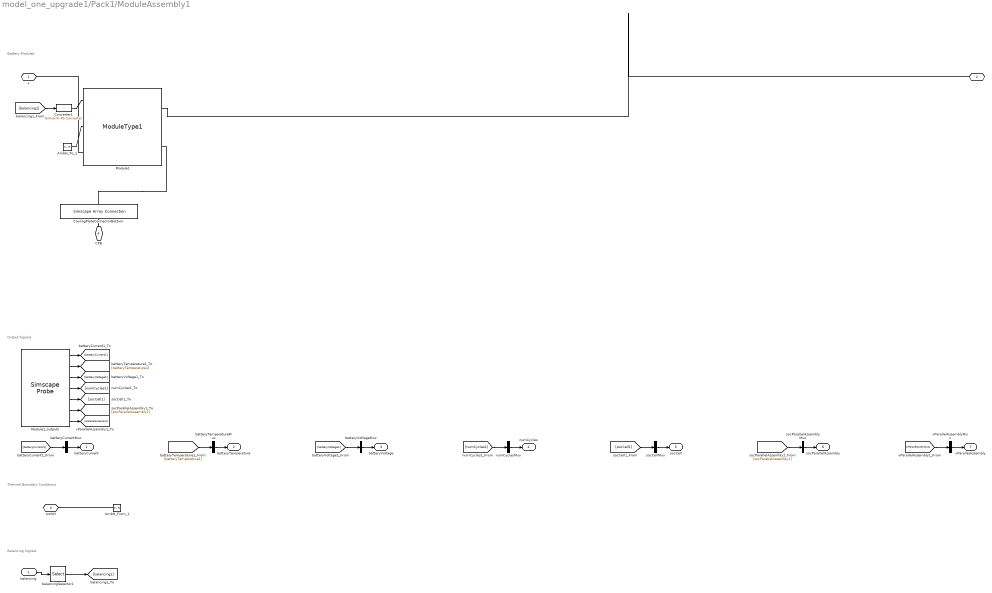
== system model_one_upgrade1/Pack1/ModuleAssembly1 ==
  note: Battery Modules
  note: Output Signals
  note: Thermal Boundary Conditions
  note: Balancing Signals
  balancing : Inport  PortDimensions=2
  AmbH_From_1 : ConnectionLabel  Label=ambH_1
  AmbH_To_1 : ConnectionLabel  Label=ambH_1
  Converter1 : nesl_utility/Simulink-PS Converter  PhysicalDomain=network_engine_domain  SubClassName=ps_input  LeftPortType=input  RightPortType=output  PseudoPeriodic=off  Frequencies=[]  NoiseDistribution=none  NoiseParameters=[]  Unit=1  AffineConversion=off  FilteringAndDerivatives=provide  SimscapeFilterOrder=1  InputFilterTimeConstant=0.001  UdotUserProvided=0
  CoolingPlateConnectorBottom : SimscapeArrayConnection  Domain=foundation.thermal.thermal  Mode=Sized Elements
  Module1 : Batteries_Pack_lib/Modules/ModuleType1  BatteryCapacityCell=2.65 A*hr  ExtrapolationMethodCell=simscape.enum.extrapolation.linear  SOCBreakpointsCell=[0, .01, .02, .03, .04, .05, .06, .07, .08, .09, .1, .11, .12, .13, .14, .15, .16, .17, .18, .19, .2, .21, .22, .23, .24, .25, .26, .27, .28, .29, .3, .31, .32, .33, .34, .35, .36, .37, .38, .39, .4, .41, .42, .43, .44, .45, .46, .47, .48, .49, .5, .51, .52, .53, .54, .55, .56, .57, .58, .59, .6, .61, .62, .63, .64, .65, .66, .67, .68, .69, .7, .71, .72, .73, .74, .75, .76, .77, .78, .79, .8, .81, .82, .83, .84, .85, .86, .87, .88, .89, .9, .91, .92, .93, .94, .95, .96, .97, .98, .99, 1]  TemperatureBreakpointsCell=[0, 25, 40, 60] degC  OpenCircuitVoltageThermalCell=[3.04339, 3.04339, 3.04339, 3.04339; 3.19969, 3.19969, 3.19969, 3.19969; 3.32733, 3.32733, 3.32733, 3.32733; 3.41897, 3.41897, 3.41897, 3.41897; 3.47789, 3.47789, 3.47789, 3.47789; 3.5189, 3.5189, 3.5189, 3.5189; 3.54757, 3.54757, 3.54757, 3.54757; 3.56926, 3.56926, 3.56926, 3.56926; 3.58543, 3.58543, 3.58543, 3.58543; 3.59715, 3.59715, 3.59715, 3.59715; 3.60656, 3.60656, 3.60656, 3.60656; 3.61458, 3.61458, 3.61458, 3.61458; 3.62125, 3.62125, 3.62125, 3.62125; 3.62859, 3.62859, 3.62859, 3.62859; 3.63585, 3.63585, 3.63585, 3.63585; 3.64117, 3.64117, 3.64117, 3.64117; 3.64677, 3.64677, 3.64677, 3.64677; 3.65281, 3.65281, 3.65281, 3.65281; 3.65754, 3.65754, 3.65754, 3.65754; 3.6622, 3.6622, 3.6622, 3.6622; 3.66686, 3.66686, 3.66686, 3.66686; 3.67118, 3.67118, 3.67118, 3.67118; 3.67547, 3.67547, 3.67547, 3.67547; 3.67953, 3.67953, 3.67953, 3.67953; 3.68333, 3.68333, 3.68333, 3.68333; 3.68679, 3.68679, 3.68679, 3.68679; 3.68929, 3.68929, 3.68929, 3.68929; 3.69163, 3.69163, 3.69163, 3.69163; 3.69398, 3.69398, 3.69398, 3.69398; 3.69633, 3.69633, 3.69633, 3.69633; 3.69868, 3.69868, 3.69868, 3.69868; 3.70108, 3.70108, 3.70108, 3.70108; 3.7035, 3.7035, 3.7035, 3.7035; 3.70592, 3.70592, 3.70592, 3.70592; 3.70834, 3.70834, 3.70834, 3.70834; 3.71076, 3.71076, 3.71076, 3.71076; 3.71334, 3.71334, 3.71334, 3.71334; 3.71599, 3.71599, 3.71599, 3.71599; 3.71889, 3.71889, 3.71889, 3.71889; 3.72198, 3.72198, 3.72198, 3.72198; 3.72508, 3.72508, 3.72508, 3.72508; 3.72817, 3.72817, 3.72817, 3.72817; 3.73126, 3.73126, 3.73126, 3.73126; 3.73436, 3.73436, 3.73436, 3.73436; 3.73745, 3.73745, 3.73745, 3.73745; 3.74054, 3.74054, 3.74054, 3.74054; 3.74364, 3.74364, 3.74364, 3.74364; 3.74686, 3.74686, 3.74686, 3.74686; 3.75011, 3.75011, 3.75011, 3.75011; 3.75346, 3.75346, 3.75346, 3.75346; 3.75768, 3.75768, 3.75768, 3.75768; 3.7621, 3.7621, 3.7621, 3.7621; 3.76652, 3.76652, 3.76652, 3.76652; 3.77094, 3.77094, 3.77094, 3.77094; 3.77575, 3.77575, 3.77575, 3.77575; 3.78058, 3.78058, 3.78058, 3.78058; 3.78546, 3.78546, 3.78546, 3.78546; 3.79147, 3.79147, 3.79147, 3.79147; 3.79777, 3.79777, 3.79777, 3.79777; 3.80409, 3.80409, 3.80409, 3.80409; 3.8104, 3.8104, 3.8104, 3.8104; 3.81672, 3.81672, 3.81672, 3.81672; 3.82303, 3.82303, 3.82303, 3.82303; 3.82935, 3.82935, 3.82935, 3.82935; 3.83618, 3.83618, 3.83618, 3.83618; 3.84344, 3.84344, 3.84344, 3.84344; 3.8508, 3.8508, 3.8508, 3.8508; 3.85816, 3.85816, 3.85816, 3.85816; 3.86553, 3.86553, 3.86553, 3.86553; 3.87289, 3.87289, 3.87289, 3.87289; 3.88052, 3.88052, 3.88052, 3.88052; 3.88833, 3.88833, 3.88833, 3.88833; 3.89603, 3.89603, 3.89603, 3.89603; 3.90423, 3.90423, 3.90423, 3.90423; 3.91256, 3.91256, 3.91256, 3.91256; 3.92124, 3.92124, 3.92124, 3.92124; 3.93029, 3.93029, 3.93029, 3.93029; 3.93933, 3.93933, 3.93933, 3.93933; 3.94837, 3.94837, 3.94837, 3.94837; 3.95788, 3.95788, 3.95788, 3.95788; 3.96788, 3.96788, 3.96788, 3.96788; 3.97854, 3.97854, 3.97854, 3.97854; 3.98931, 3.98931, 3.98931, 3.98931; 4.00008, 4.00008, 4.00008, 4.00008; 4.01149, 4.01149, 4.01149, 4.01149; 4.02304, 4.02304, 4.02304, 4.02304; 4.03459, 4.03459, 4.03459, 4.03459; 4.04614, 4.04614, 4.04614, 4.04614; 4.05768, 4.05768, 4.05768, 4.05768; 4.06947, 4.06947, 4.06947, 4.06947; 4.08184, 4.08184, 4.08184, 4.08184; 4.09422, 4.09422, 4.09422, 4.09422; 4.1067, 4.1067, 4.1067, 4.1067; 4.11982, 4.11982, 4.11982, 4.11982; 4.1326, 4.1326, 4.1326, 4.1326; 4.14615, 4.14615, 4.14615, 4.14615; 4.15754, 4.15754, 4.15754, 4.15754; 4.16699, 4.16699, 4.16699, 4.16699; 4.17222, 4.17222, 4.17222, 4.17222; 4.18119, 4.18119, 4.18119, 4.18119; 4.30838, 4.30838, 4.30838, 4.30838] V  VoltageRangeCell=[2.7, Inf] V  ResistanceSOCBreakpointsCell=[0, .01, .02, .03, .04, .05, .06, .07, .08, .09, .1, .11, .12, .13, .14, .15, .16, .17, .18, .19, .2, .21, .22, .23, .24, .25, .26, .27, .28, .29, .3, .31, .32, .33, .34, .35, .36, .37, .38, .39, .4, .41, .42, .43, .44, .45, .46, .47, .48, .49, .5, .51, .52, .53, .54, .55, .56, .57, .58, .59, .6, .61, .62, .63, .64, .65, .66, .67, .68, .69, .7, .71, .72, .73, .74, .75, .76, .77, .78, .79, .8, .81, .82, .83, .84, .85, .86, .87, .88, .89, .9, .91, .92, .93, .94, .95, .96, .97, .98, .99, 1]  ResistanceTemperatureBreakpointsCell=[0, 25, 40, 60] degC  R0ThermalCell=[.10009, .04577, .01007, .01632; .14613, .0693, .01231, .013; .1823, .0871, .02576, .02712; .20605, .0981, .03749, .03657; .21852, .10274, .04624, .03593; .22481, .10473, .05239, .04275; .22685, .1047, .05724, .04532; .22648, .10401, .05969, .04893; .22421, .1029, .06023, .05216; .2204, .10084, .06022, .05386; .2158, .09855, .06061, .05477; .21072, .0961, .06053, .05519; .20518, .09374, .05997, .05515; .19986, .0923, .05976, .05534; .19452, .09098, .06051, .05551; .19005, .08942, .06059, .055; .18649, .08829, .06076, .05491; .18308, .08779, .06108, .05531; .17921, .08711, .06095, .05525; .17533, .08642, .06116, .05516; .17188, .08573, .06162, .05537; .16959, .08504, .06197, .05562; .16728, .08435, .0623, .05586; .16489, .08362, .06255, .05603; .16242, .08285, .06272, .0561; .15982, .0821, .06284, .05605; .15726, .08136, .06262, .05568; .15524, .08067, .06235, .05525; .15322, .07998, .06208, .05483; .1512, .07929, .06181, .05441; .14918, .07859, .06154, .05399; .14718, .07791, .06129, .05359; .14518, .07723, .06105, .05316; .14319, .07655, .06062, .05273; .14155, .07588, .06014, .0523; .14028, .0752, .05965, .05186; .13906, .07463, .05921, .05149; .13787, .07414, .0588, .05114; .13676, .07372, .05848, .05087; .13572, .07333, .05823, .05067; .13469, .07295, .05797, .05047; .13365, .07256, .05771, .05028; .13261, .07218, .05746, .0497; .13157, .07179, .0572, .04908; .13053, .07141, .05667, .04845; .12949, .07102, .05603, .04793; .1286, .07064, .05539, .04744; .12808, .07034, .05479, .04699; .12757, .07007, .0542, .04656; .1271, .06981, .05364, .04615; .12693, .06973, .05339, .04605; .12682, .0697, .0532, .04601; .12672, .06966, .05301, .04589; .12661, .06963, .05283, .04564; .12664, .06966, .05277, .04553; .12668, .06969, .05273, .04542; .12673, .06974, .0527, .04507; .12716, .07, .05306, .04491; .12758, .07016, .053, .04485; .128, .07032, .0529, .04479; .12841, .07047, .0528, .04474; .12883, .07062, .0527, .04468; .12925, .07078, .05261, .04463; .12967, .07093, .05251, .04457; .13027, .07117, .05259, .04469; .13101, .0715, .05282, .04497; .13204, .07186, .05308, .04484; .13321, .07221, .05335, .04472; .13439, .07256, .0532, .04459; .13557, .07292, .05301, .04446; .13684, .07332, .05292, .04443; .13817, .07375, .05288, .04428; .13946, .0741, .05281, .04407; .14091, .07448, .05291, .04404; .14233, .07489, .05306, .04405; .14388, .07535, .05333, .04418; .14556, .07584, .05372, .04444; .14723, .07633, .05411, .0447; .14891, .07682, .0545, .04496; .15108, .07759, .05506, .04537; .15372, .07866, .05578, .04596; .15659, .07988, .05673, .04678; .1595, .08112, .0574, .04703; .16241, .08236, .05796, .04728; .16616, .08368, .05874, .04774; .17134, .08499, .05957, .04825; .17651, .0863, .0604, .04877; .18169, .08761, .06123, .04928; .18774, .08891, .06206, .04979; .19646, .09039, .06297, .05038; .20538, .09225, .06408, .05118; .2143, .09411, .0652, .05198; .22836, .09597, .06593, .05281; .24309, .09796, .06644, .05348; .25899, .0995, .06683, .05394; .28056, .10104, .06749, .05466; .30009, .10043, .0674, .05464; .31508, .09826, .06607, .05332; .32861, .09216, .06054, .05002; .31916, .08512, .05631, .04686; .33322, .00997, .09284, .03396] Ohm  BatteryThermalMassCell=44.1 J/K  CoolantResistance=1.2 K/W  AmbientResistance=25 K/W  InterCellThermalResistance=1 K/W  InterParallelAssemblyThermalResistance=1 K/W  CellBalancingClosedResistance=0.01 Ohm  CellBalancingOpenConductance=1e-8 1/Ohm  CellBalancingThreshold=0.5  CellBalancingResistance=50 Ohm  P=2  S=2  NumInterCellThermalConnections=2  NumInterParallelAssemblyThermalConnections=4  InterParallelAssemblyConnectionsMapping=[1, 1, 1, 1; 2, 2, 2, 2]  InterParallelAssemblyCellConnectionsMapping=[1, 1, 2, 2; 1, 2, 1, 2]  InterCellConnectionsMapping=[1, 1; 2, 2]  socCell_specify=on  socCell_priority=High  socCell=repmat(0.8, 4, 1)  socCell_nominal_specify=off  socCell_nominal_value=1  socCell_nominal_unit=1  batteryVoltage_specify=off  batteryVoltage_priority=None  batteryVoltage=repmat(0, 4, 1) V  batteryVoltage_nominal_specify=off  batteryVoltage_nominal_value=1  batteryVoltage_nominal_unit=V  batteryCurrent_specify=off  batteryCurrent_priority=None  batteryCurrent=repmat(0, 4, 1) A  batteryCurrent_nominal_specify=off  batteryCurrent_nominal_value=1  batteryCurrent_nominal_unit=A  numCycles_specify=off  numCycles_priority=High  numCycles=repmat(0, 4, 1)  numCycles_nominal_specify=off  numCycles_nominal_value=1  numCycles_nominal_unit=1  batteryTemperature_specify=off  batteryTemperature_priority=High  batteryTemperature=repmat(298.15, 4, 1) K  batteryTemperature_nominal_specify=off  batteryTemperature_nominal_value=1  batteryTemperature_nominal_unit=K  vParallelAssembly_specify=off  vParallelAssembly_priority=None  vParallelAssembly=repmat(0, 2, 1) V  vParallelAssembly_nominal_specify=off  vParallelAssembly_nominal_value=1  vParallelAssembly_nominal_unit=V  socParallelAssembly_specify=on  socParallelAssembly_priority=None  socParallelAssembly=repmat(0.8, 2, 1)  socParallelAssembly_nominal_specify=off  socParallelAssembly_nominal_value=1  socParallelAssembly_nominal_unit=1
      settings: InternalSimscapePortConfiguration="{\"Bottom\":[{\"id\":\"n\",\"label\":\"-\",\"type\":\"foundation.electrical.electrical\"},{\"id\":\"BottomExtClnt\",\"label\":\"CPB\",\"type\":\"foundation.thermal.thermal\"}],\"Left\":[{\"id\":\"enableCellBalancing\",\"label\":\"CB\",\"type\":\"input\"},{\"id\":\"AmbH\",\"label\":\"AmbH\",\"type\":\"foundation.thermal.thermal\"}],\"Right\":[],\"Top\":[{\"id\":\"p\",\"label\":\"+\",\"type\":\"foundation.electrical.electrical\"}]}"
  Module1_outputs : SimscapeProbe  BoundBlock=151  Variables="{\"batteryCurrent\":{\"Probing\":\"ON\"},\"batteryTemperature\":{\"Probing\":\"ON\"},\"batteryVoltage\":{\"Probing\":\"ON\"},\"numCycles\":{\"Probing\":\"ON\"},\"socCell\":{\"Probing\":\"ON\"},\"socParallelAssembly\":{\"Probing\":\"ON\"},\"vParallelAssembly\":{\"Probing\":\"ON\"}}"
  balancingSelector1 : Selector  InputPortWidth=2  IndexOptions=Index vector (dialog)  Indices="[1  2]"  OutputSizes=1
  batteryCurrentMux : Mux  Inputs=1
  batteryTemperatureMux : Mux  Inputs=1
  batteryVoltageMux : Mux  Inputs=1
  numCyclesMux : Mux  Inputs=1
  socCellMux : Mux  Inputs=1
  socParallelAssemblyMux : Mux  Inputs=1
  vParallelAssemblyMux : Mux  Inputs=1
  + : PMIOPort  Side=Left
  - : PMIOPort  Port=2  Side=Right
  AmbH : PMIOPort  Port=3  Side=Right  ConnectionType=Connection: foundation.thermal.thermal
  CPB : PMIOPort  Port=4  Side=Right  ConnectionType=Connection: foundation.thermal.thermal
  batteryCurrent : Outport
  batteryTemperature : Outport  Port=2
  batteryVoltage : Outport  Port=3
  numCycles : Outport  Port=4
  socCell : Outport  Port=5
  socParallelAssembly : Outport  Port=6
  vParallelAssembly : Outport  Port=7
  wires:
  Module1_outputs/1 -> [batteryCurrent1]
  batteryCurrentMux/1 -> batteryCurrent/1
  [batteryCurrent1] -> batteryCurrentMux/1
  Module1_outputs/2 -> [batteryTemperature1]
  batteryTemperatureMux/1 -> batteryTemperature/1
  [batteryTemperature1] -> batteryTemperatureMux/1
  Module1_outputs/3 -> [batteryVoltage1]
  batteryVoltageMux/1 -> batteryVoltage/1
  [batteryVoltage1] -> batteryVoltageMux/1
  Module1_outputs/4 -> [numCycles1]
  numCyclesMux/1 -> numCycles/1
  [numCycles1] -> numCyclesMux/1
  Module1_outputs/5 -> [socCell1]
  socCellMux/1 -> socCell/1
  [socCell1] -> socCellMux/1
  Module1_outputs/6 -> [socParallelAssembly1]
  socParallelAssemblyMux/1 -> socParallelAssembly/1
  [socParallelAssembly1] -> socParallelAssemblyMux/1
  Module1_outputs/7 -> [vParallelAssembly1]
  vParallelAssemblyMux/1 -> vParallelAssembly/1
  [vParallelAssembly1] -> vParallelAssemblyMux/1
  [balancing1] -> Converter1/1
  balancing/1 -> balancingSelector1/1
  balancingSelector1/1 -> [balancing1]
  connections:
  Module1/LConn3 -- +/RConn1
  Module1/RConn1 -- -/RConn1
  Converter1/RConn1 -- Module1/LConn1
  AmbH_To_1/LConn1 -- Module1/LConn2
  AmbH_From_1/LConn1 -- AmbH/RConn1
  CoolingPlateConnectorBottom/LConn1 -- Module1/RConn2
  CoolingPlateConnectorBottom/RConn1 -- CPB/RConn1
